simulink model "TD2_Ex2_sim"  (R2022a)
settings: Solver=VariableStepAuto  StartTime=0.0  StopTime=10.0  RelTol=1e-3
undefined symbols (not defined in the file): A, B, C
settings Model: Creator=CS  LastModifiedBy=CS

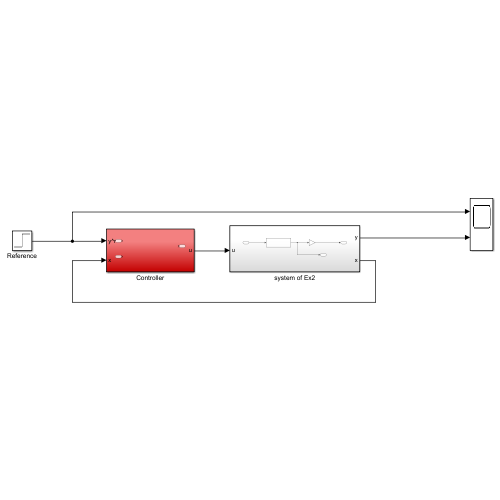
[thumbnail: Simulink's stored preview of the top-level diagram]
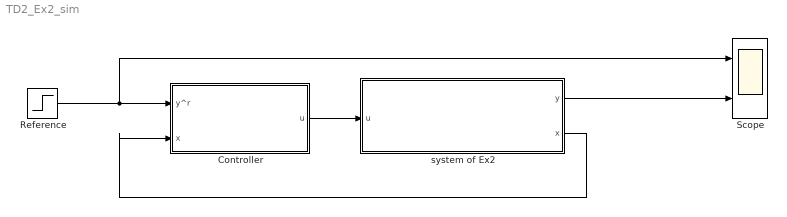
== system TD2_Ex2_sim ==
  Controller : Subsystem
  Reference : Step  SampleTime=0
  Scope : Scope  NumInputPorts=2
  system of Ex2 : Subsystem
  wires:
  system of Ex2/1(y) -> Scope/2
  Reference/1 -> Controller/1(y^r), Scope/1
  system of Ex2/2(x) -> Controller/2(x)
  Controller/1(u) -> system of Ex2/1(u)

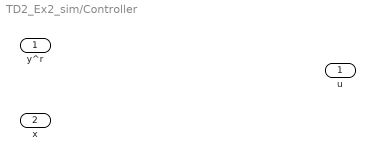
== system TD2_Ex2_sim/Controller ==
  y^r : Inport
  x : Inport  Port=2
  u : Outport

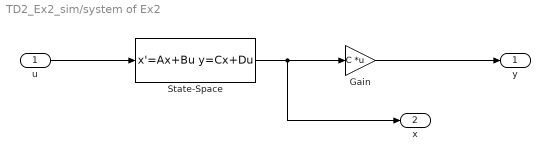
== system TD2_Ex2_sim/system of Ex2 ==
  u : Inport
  Gain : Gain  Gain=C  Multiplication=Matrix(K*u) (u vector)
  State-Space : StateSpace  A=A  B=B  C=eye(3)  D=zeros(3,1)  InitialCondition=0
  y : Outport
  x : Outport  Port=2
  wires:
  u/1 -> State-Space/1
  State-Space/1 -> x/1, Gain/1
  Gain/1 -> y/1
